simulink model "AssembledTEST1"  (R2016b)
settings: Solver=VariableStepAuto  StartTime=0.0  StopTime=60  RelTol=1e-3
values from neighbouring files (symbols this model uses):
  ail_data = [ ... (first row only)    [lookup_init.m]
  Ap = pi * (D^2)/4    (= 5.69167367599)    [constants_init.m]
  Aw = 10.0    (= 10)    [constants_init.m]
  b = 15.85    [constants_init.m]
  beta0_data = [ ... (first row only)    [lookup_init.m]
  c0 = 2.3774    [constants_init.m]
  c_i = 1.847    [constants_init.m]
  cdrag_data = [ ... (first row only)    [lookup_init.m]
  clean_wing_data = [ ... (first row only)    [lookup_init.m]
  crt = 1.6764    [constants_init.m]
  CT_data = [ ... (first row only)    [lookup_init.m]
  D = 2.692    [constants_init.m]
  D0q_10 = 0.0778    [constants_init.m]
  D0q_20 = 0.2634    [constants_init.m]
  D0q_35 = 0.7099    [constants_init.m]
  DCDi_data = [ ... (first row only)    [lookup_init.m]
  DCM0b = -0.188    [constants_init.m]
  Deh_f_on_data = [ ... (first row only)    [lookup_init.m]
  Deh_on_data = [ ... (first row only)    [lookup_init.m]
  df = 1.981    [constants_init.m]
  DOWN_0 = HP * F2M    (= 1830.0192)    [InitialiseJ31.m]    (also in Trim.m = -xtrim(12))
  Dqhq_data = [ ... (first row only)    [lookup_init.m]
  e0 = d2r(2.0)    [constants_init.m]
  e_data10 = [ ... (first row only)    [lookup_init.m]
  e_data20 = [ ... (first row only)    [lookup_init.m]
  e_data35 = [ ... (first row only)    [lookup_init.m]
  EAST_0 = 0.0    (= 0)    [InitialiseJ31.m]    (also in Trim.m = xtrim(11))
  elaw_0 = -7.50225e+2    (= -750.225)    [constants_init.m]
  elaw_1 = 8.98698    [constants_init.m]
  elaw_2 = -6.94240e-3    (= -0.0069424)    [constants_init.m]
  FLAP = 0    [InitialiseJ31.m]
  flaps_lift_data = [ ... (first row only)    [lookup_init.m]
  flaps_moment_data = [ ... (first row only)    [lookup_init.m]
  flaps_tail_data = [ ... (first row only)    [lookup_init.m]
  flaps_wing_data = [ ... (first row only)    [lookup_init.m]
  fmc_data = [ ... (first row only)    [lookup_init.m]
  fmf_data = [ ... (first row only)    [lookup_init.m]
  fmn_data = [ ... (first row only)    [lookup_init.m]
  fus_data = [ ... (first row only)    [lookup_init.m]
  gamma_t = 0.578    [constants_init.m]
  h_data10 = [ ... (first row only)    [lookup_init.m]
  h_data20 = [ ... (first row only)    [lookup_init.m]
  h_data35 = [ ... (first row only)    [lookup_init.m]
  INERTIA = [IXX,IXY,IXZ;IXY,IYY,IYZ;IXZ,IYZ,IZZ]    [InitialiseJ31.m]
  it = d2r(-2.3)    [constants_init.m]
  iw = d2r(1.33)    [constants_init.m]
  Iwn2 = 0.636    [constants_init.m]
  J_W = 1.26    [constants_init.m]
  K1_data = [ ... (first row only)    [lookup_init.m]
  k1f_data = [ ... (first row only)    [lookup_init.m]
  k_data = [ ... (first row only)    [lookup_init.m]
  L_r0_10f = -0.0096    [constants_init.m]
  L_r0_20f = -0.0180    (= -0.018)    [constants_init.m]
  L_r0_35f = -0.0245    [constants_init.m]
  l_t = 11.6205 - 5.6642    (= 5.9563)    [constants_init.m]
  ld_data = [ ... (first row only)    [lookup_init.m]
  Lt = 4.686    [constants_init.m]
  Lt_dash = 247.1 * 0.3048/12    (= 6.27634)    [constants_init.m]
  Lv_b = -0.00145    [constants_init.m]
  Lv_h = 0.0445    [constants_init.m]
  Lv_n = 0.0165    [constants_init.m]
  mac = 1.716    [constants_init.m]
  mach_ffr = 0.4158    [constants_init.m]
  mach_pow = 0.7984    [constants_init.m]
  n = 1591/60    (= 26.5166666667)    [constants_init.m]
  NORTH_0 = 0.0    (= 0)    [InitialiseJ31.m]    (also in Trim.m = xtrim(10))
  Nr_b = -0.0060    (= -0.006)    [constants_init.m]
  Nv_n = -0.0005    [constants_init.m]
  Nv_wb = -0.0719    [constants_init.m]
  P_0 = 0.0    (= 0)    [InitialiseJ31.m]    (also in Trim.m = xtrim(4))
  pdrag_data = [ ... (first row only)    [lookup_init.m]
  PHI_0 = xtrim(7)    [Trim.m]
  piAt = At * pi    (= 17.5929188601)    [constants_init.m]
  piAw = Aw * pi    (= 31.4159265359)    [constants_init.m]
  PSI_0 = xtrim(9)    [Trim.m]
  Q_0 = 0.0    (= 0)    [InitialiseJ31.m]    (also in Trim.m = xtrim(5))
  R2D = 180/pi    (= 57.2957795131)    [InitialiseJ31.m]
  R_0 = 0.0    (= 0)    [InitialiseJ31.m]    (also in Trim.m = xtrim(6))
  s_e = 0.0954    [constants_init.m]
  side_data = [ ... (first row only)    [lookup_init.m]
  sideforce_data = [ ... (first row only)    [lookup_init.m]
  Sit = 1.874    [constants_init.m]
  Sn = 0.552    [constants_init.m]
  Sref = (pi/4) * df^2    (= 3.08218592191)    [constants_init.m]
  St = 7.785    [constants_init.m]
  Sw = 25.084    [constants_init.m]
  tail_data = [ ... (first row only)    [lookup_init.m]
  THETA_0 = xtrim(8)    [Trim.m]
  U_0 = xtrim(1)    [Trim.m]
  upwash_clean = [ ... (first row only)    [lookup_init.m]
  upwash_flaps = [ ... (first row only)    [lookup_init.m]
  V_0 = xtrim(2)    [Trim.m]
  vortex_drag_factors = [ ... (first row only)    [lookup_init.m]
  W_0 = xtrim(3)    [Trim.m]
  X_ci = ((223 - 140)*0.3048/12) - Xp_dash    (= 0.09144)    [constants_init.m]
  xacf = -6.653    [constants_init.m]
  xacn = (223 - 197.3)*0.3048/12    (= 0.65278)    [constants_init.m]
  xb0 = c0 * xb0_c0    (= 0.5895952)    [constants_init.m]
  xcit = -l_t - ycit * sin(d2r(11.31)) - (0.981/4)    [constants_init.m]
  Xp_dash = 79.4  * 0.3048/12    (= 2.01676)    [constants_init.m]
  xyz_p = [140.0*0.3048/12;-107.0*0.3048/12;11.5*0.3048/12]    [constants_init.m]
  xyz_s = [140.0*0.3048/12; 107.0*0.3048/12;11.5*0.3048/12]    [constants_init.m]
  ycit = 2.306    [constants_init.m]
  Yr_b = -0.0283    [constants_init.m]
  Yv_n = -0.0458    [constants_init.m]
  Yv_wb = -0.2627    [constants_init.m]
  Z_ht = 11.5*0.3048/12 - zact    (= 1.7271)    [constants_init.m]
  zacf = -1.741    [constants_init.m]
  zacn = 11.5*0.3048/12    (= 0.2921)    [constants_init.m]
  zact = -1.435    [constants_init.m]
  zacw = 0.929 - (3.307 * tan(d2r(7)))    [constants_init.m]
  Zt_dash = 12.0  * 0.3048/12    (= 0.3048)    [constants_init.m]
undefined symbols (not defined in the file or in its folder): CG, MASS
libraries: aerolibasang x3, aerolibatmos2 x1
(part 2 of 5)

== system AssembledTEST1/Subsystem/Longitudinal Aerodynamics/Get Nacelles XZM ==
  In2 : Inport
  In1 : Inport  Port=2
  Bus Selector : BusSelector  OutputSignals=alpha_b,q_bar,Flap,Mach
  Constant : Constant  Value=xacn
  Constant1 : Constant  Value=zacn
  Constant2 : Constant  Value=0
  Constant6 : Constant  Value=mac
  Constant7 : Constant  Value=Sw
  Get XZM : Subsystem
      mask Display:
      | port_label('input',1,'lift [N]')
      | port_label('input',2,'drag [N]')
      | port_label('input',3,'\alpha [rad]','texmode','on')
      | port_label('input',4,'M [Nm]','texmode','on')
      | port_label('input',5,'x_{ac} [m]','texmode','on')
      | port_label('input',6,'z_{ac} [m]','texmode','on')
      | port_label('output',1,'X [N]')
      | port_label('output',2,'Z [N]')
      | port_label('output',3,'M [Nm]')
  Product7 : Product  Inputs=5  RndMeth=Zero
  Subsystem : Subsystem
      mask Display:
      | port_label('output',1,'(C_{m\alpha})_{n(\epsilon)}','texmode','on')
      | port_label('input',1,'Flap')
      | port_label('input',2,'Mach')
  Out1 : Outport
  Out2 : Outport  Port=2
  Out3 : Outport  Port=3
  wires:
  Get XZM/1(X) -> Out1/1
  In1/1 -> Get XZM/2(D)
  Get XZM/2(Z) -> Out2/1
  Get XZM/3(M) -> Out3/1
  Constant1/1 -> Get XZM/6(z)
  Constant/1 -> Get XZM/5(x)
  In2/1 -> Bus Selector/1
  Bus Selector/1 -> Get XZM/3(alpha), Product7/1  "<alpha_b>"
  Constant6/1 -> Product7/2
  Constant7/1 -> Product7/3
  Constant2/1 -> Get XZM/1(L)
  Bus Selector/2 -> Product7/4  "<q_bar>"
  Bus Selector/3 -> Subsystem/1(In2)  "<Flap>"
  Bus Selector/4 -> Subsystem/2(In1)  "<Mach>"
  Subsystem/1(Out1) -> Product7/5
  Product7/1 -> Get XZM/4(M0)

== system AssembledTEST1/Subsystem/Longitudinal Aerodynamics/Get Tail XZM ==
  In1 : Inport
  In2 : Inport  Port=2
  In3 : Inport  Port=3
  In4 : Inport  Port=4
  In5 : Inport  Port=5
  Bus Selector : BusSelector  OutputSignals=Mach,q_bar,Elevator
  Constant1 : Constant  Value=-0.652
  Constant13 : Constant  Value=zact
  Constant2 : Constant  Value=Sw
  Constant3 : Constant  Value=mac
  Get XZM : Subsystem
      mask Display:
      | port_label('input',1,'lift [N]')
      | port_label('input',2,'drag [N]')
      | port_label('input',3,'\alpha [rad]','texmode','on')
      | port_label('input',4,'M_0 [Nm]','texmode','on')
      | port_label('input',5,'x_{ac} [m]','texmode','on')
      | port_label('input',6,'z_{ac} [m]','texmode','on')
      | port_label('output',1,'X [N]')
      | port_label('output',2,'Z [N]')
      | port_label('output',3,'M [Nm]')
  Product1 : Product  Inputs=6  RndMeth=Zero
  get kf : Lookup  InputValues=tail_data(:,1)  Table=tail_data(:,6)
  Out1 : Outport
  Out2 : Outport  Port=2
  Out3 : Outport  Port=3
  wires:
  Constant13/1 -> Get XZM/6(z)
  In1/1 -> Get XZM/1(L)
  Get XZM/1(X) -> Out1/1
  In2/1 -> Get XZM/2(D)
  In3/1 -> Get XZM/3(alpha)
  Get XZM/2(Z) -> Out2/1
  In5/1 -> Get XZM/5(x)
  Get XZM/3(M) -> Out3/1
  In4/1 -> Bus Selector/1
  Bus Selector/1 -> get kf/1  "<Mach>"
  get kf/1 -> Product1/1
  Bus Selector/2 -> Product1/2  "<q_bar>"
  Bus Selector/3 -> Product1/3  "<Elevator>"
  Constant1/1 -> Product1/4
  Constant2/1 -> Product1/5
  Constant3/1 -> Product1/6
  Product1/1 -> Get XZM/4(M0)

== system AssembledTEST1/Subsystem/Longitudinal Aerodynamics/Get Wing & Tail Lift ==
  Flap : Inport
  Mach : Inport  Port=2
  V : Inport  Port=3
  aoa : Inport  Port=4
  qbar : Inport  Port=5
  q : Inport  Port=6
  xcg : Inport  Port=7
  wdot : Inport  Port=8
  Elevator : Inport  Port=9
  Constant : Constant
  Terminator{,1..3} (4 alike) : Terminator
  get_tail_lift : Subsystem
      mask help:
      | This subsystem determines the lift and angle of attack for the tailplane at the cacluated wing angle of attack (aoa_w)  and Mach Number for the given Elevator angle. Uses the method given in ESDU 80020 and ESDU 89029. It includes modification of the incidence with pitch rate and vertical acceleration.
      |
      | Author: A Cooke Date: 24 Mar 05, modified 29 Mar 05, 8 Mar 07, 12 Sep 07
  get_wing_lift : Subsystem
      mask help:
      | This subsystem determines the lift for the wing/body combination at the specified body angle of attack (aoa), Mach Number and dynamic pressure  (qbar) for the given flap setting (Flap). Uses the method given in ESDU 96003.  It includes modification of the incidence with pitch rate.
      |
      | Author: A Cooke Date: 23 Feb 05, modified 29 Mar 05, 1 Aug 06, 8 Mar 07
  get_wing_lift_basic : Subsystem
      mask help:
      | This subsystem determines the lift for the wing/body combination at the specified body angle of attack (aoa), Mach Number and dynamic pressure  (qbar) for the given flap setting (Flap). Uses the method given in ESDU 96003.  It includes modification of the incidence with pitch rate.
      |
      | Author: A Cooke Date: 23 Feb 05, modified 29 Mar 05, 1 Aug 06, 8 Mar 07
  wng_lift : Outport
  CLw : Outport  Port=2
  aoa_w : Outport  Port=3
  xac_w : Outport  Port=4
  CLt : Outport  Port=5
  tail_lift : Outport  Port=6
  aoa_t : Outport  Port=7
  a1t : Outport  Port=8
  downwash : Outport  Port=9
  xac_t : Outport  Port=10
  CLb : Outport  Port=11
  alpha0 : Outport  Port=12
  wires:
  Flap/1 -> get_wing_lift/1(Flap), get_tail_lift/11(Flap)
  Mach/1 -> get_tail_lift/1(Mach), get_wing_lift_basic/2(Mach), get_wing_lift/2(Mach)
  V/1 -> get_wing_lift/3(V), get_tail_lift/3(V), get_wing_lift_basic/3(V)
  aoa/1 -> get_wing_lift/4(aoa), get_wing_lift_basic/4(aoa)
  qbar/1 -> get_wing_lift/5(qbar), get_tail_lift/2(qbar), get_wing_lift_basic/5(qbar)
  get_wing_lift/1(wing_lift) -> wng_lift/1
  q/1 -> get_wing_lift/6(q), get_tail_lift/4(q), get_wing_lift_basic/6(q)
  xcg/1 -> get_wing_lift/7(xcg), get_tail_lift/5(xcg), get_wing_lift_basic/7(xcg)
  get_wing_lift/2(CL) -> CLw/1
  get_wing_lift/3(aoa_w) -> aoa_w/1, get_tail_lift/6(aoa_w)
  get_wing_lift/4(alpha0) -> get_tail_lift/9(alpha0), alpha0/1
  get_tail_lift/1(aoa_t) -> aoa_t/1
  get_tail_lift/2(CLt) -> CLt/1
  get_tail_lift/3(tail_lift) -> tail_lift/1
  wdot/1 -> get_tail_lift/7(wdot)
  Elevator/1 -> get_tail_lift/8(Elevator)
  get_tail_lift/4(a1t) -> a1t/1
  get_tail_lift/5(e) -> downwash/1
  get_tail_lift/6(xac_t) -> xac_t/1
  get_wing_lift/5(xac_w) -> get_tail_lift/10(xac_w), xac_w/1
  Constant/1 -> get_wing_lift_basic/1(Flap)
  get_wing_lift_basic/1(wing_lift) -> Terminator/1
  get_wing_lift_basic/2(CL) -> CLb/1
  get_wing_lift_basic/3(aoa_w) -> Terminator1/1
  get_wing_lift_basic/4(alpha0) -> Terminator2/1
  get_wing_lift_basic/5(xac_w) -> Terminator3/1

== system AssembledTEST1/Subsystem/Longitudinal Aerodynamics/Get Wing XZM ==
  In1 : Inport
  In2 : Inport  Port=2
  In3 : Inport  Port=3
  In4 : Inport  Port=4
  In5 : Inport  Port=5
  Bus Selector3 : BusSelector  OutputSignals=Mach,Flap,q_bar
  Constant9 : Constant  Value=zacw
  Get XZM : Subsystem
      mask Display:
      | port_label('input',1,'drag [N]')
      | port_label('input',2,'lift [N]')
      | port_label('input',3,'\alpha [rad]','texmode','on')
      | port_label('input',4,'M_0 [Nm]','texmode','on')
      | port_label('input',5,'x_{ac} [m]','texmode','on')
      | port_label('input',6,'z_{ac} [m]','texmode','on')
      | port_label('output',1,'X [N]')
      | port_label('output',2,'Z [N]')
      | port_label('output',3,'M [Nm]')
  get_M0w : Subsystem
  Out1 : Outport
  Out2 : Outport  Port=2
  Out3 : Outport  Port=3
  wires:
  Bus Selector3/3 -> get_M0w/3(qbar)  "<q_bar>"
  Bus Selector3/2 -> get_M0w/2(Flap)  "<Flap>"
  Bus Selector3/1 -> get_M0w/1(Mach)  "<Mach>"
  get_M0w/1(M0) -> Get XZM/4(M0)
  Constant9/1 -> Get XZM/6(z)
  In3/1 -> Get XZM/3(alpha)
  In1/1 -> Get XZM/1(D)
  Get XZM/1(X) -> Out1/1
  In2/1 -> Get XZM/2(L)
  Get XZM/2(Z) -> Out2/1
  In4/1 -> Bus Selector3/1
  In5/1 -> Get XZM/5(x)
  Get XZM/3(M) -> Out3/1

== system AssembledTEST1/Subsystem/Longitudinal Aerodynamics/get_CDvwbasic ==
  aoa_w : Inport
  flap : Inport  Port=2
  CLw : Inport  Port=3
  Mach : Inport  Port=4
  Add4 : Sum  Inputs=+++
  Constant2 : Constant  Value=piAw
  Divide : Product  Inputs=*/
  Fcn1 : Fcn  Expr=u(1)^2
  Fcn2 : Fcn  Expr=u(1)^2
  Product3 : Product  RndMeth=Zero
  Product4 : Product  RndMeth=Zero
  Product5 : Product  Inputs=3  RndMeth=Zero
  get_CL1 : Sum  Inputs=+-
  get_DelCL0tw : Subsystem
  get_k1 : Lookup2D  RowIndex=aw_ords  ColumnIndex=Mach_ords  Table=k_data
  get_k1f : Lookup  InputValues=k1f_data(:,1)  Table=k1f_data(:,2)
  get_kf : Subsystem
  r2d : Gain  Gain=180/pi
  CDvw : Outport
  wires:
  get_DelCL0tw/1(DelCL0tw) -> get_CL1/2, Fcn2/1, Product5/2
  get_CL1/1 -> Fcn1/1, Product5/3
  Fcn2/1 -> Product3/1
  get_kf/1(kf) -> Product3/2
  Fcn1/1 -> Product4/1
  get_k1/1 -> Product4/2
  get_k1f/1 -> Product5/1
  Product5/1 -> Add4/1
  Product4/1 -> Add4/2
  Product3/1 -> Add4/3
  Add4/1 -> Divide/1
  Constant2/1 -> Divide/2
  flap/1 -> get_DelCL0tw/1(flap), get_kf/1(flap)
  Mach/1 -> get_DelCL0tw/2(Mach), get_kf/2(Mach), get_k1/2
  aoa_w/1 -> get_k1f/1, r2d/1
  Divide/1 -> CDvw/1
  CLw/1 -> get_CL1/1
  r2d/1 -> get_k1/1

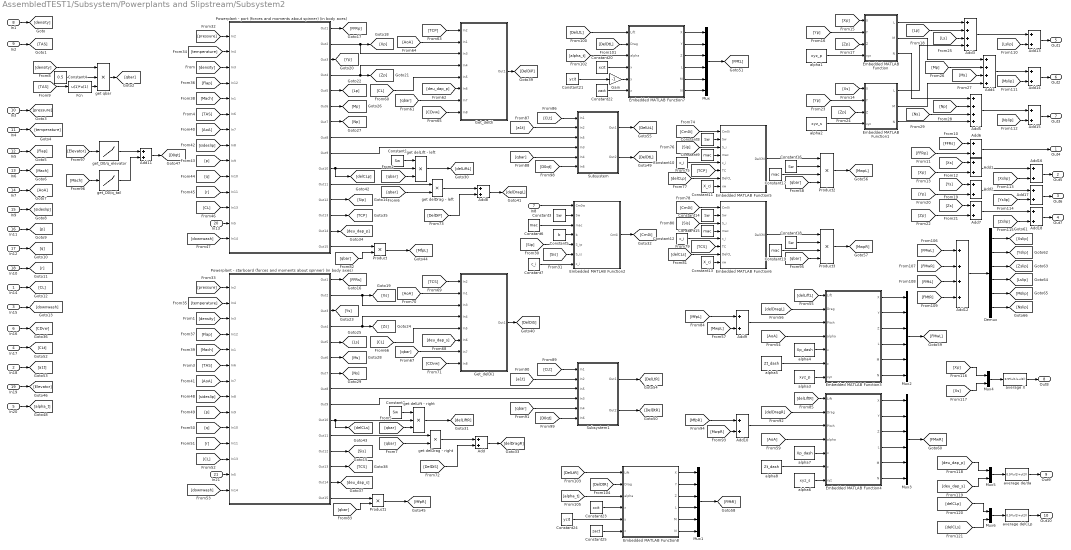
== system AssembledTEST1/Subsystem/Powerplants and Slipstream/Subsystem2 ==
  In14 : Inport
  In18 : Inport  Port=2
  In15 : Inport  Port=3
  In17 : Inport  Port=4
  In20 : Inport  Port=5
  In16 : Inport  Port=6
  In8 : Inport  Port=7
  In1 : Inport  Port=8
  In2 : Inport  Port=9
  In3 : Inport  Port=10
  In4 : Inport  Port=11
  In5 : Inport  Port=12
  In6 : Inport  Port=13
  In7 : Inport  Port=14
  In9 : Inport  Port=15
  In11 : Inport  Port=16
  In12 : Inport  Port=17
  In10 : Inport  Port=18
  In19 : Inport  Port=19
  In13 : Inport  Port=20
  In21 : Inport  Port=21
  Add{,1..2,6..11,13..18} (15 alike) : Sum
  Add{3..5,12} (4 alike) : Sum  Inputs=++++
  Constant{1..3,8,14,16,18} (7 alike) : Constant  Value=Sw
  Constant10 : Constant  Value=c_i
  Constant11 : Constant  Value=X_ci
  Constant12 : Constant  Value=c_i
  Constant13 : Constant  Value=X_ci
  Constant{6,9,15,17,19} (5 alike) : Constant  Value=mac
  Constant20 : Constant  Value=xcit
  Constant21 : Constant  Value=ycit
  Constant22 : Constant  Value=zact
  Constant23 : Constant  Value=xcit
  Constant24 : Constant  Value=ycit
  Constant25 : Constant  Value=zact
  Constant4 : Constant  Value=0.5
  Constant5 : Constant  Value=b
  Constant7 : Constant  Value=c_i
  Demux : Demux  Outputs=6
  Embedded MATLAB Function : MATLAB Function  TreatAsAtomicUnit=on
  Embedded MATLAB Function1 : MATLAB Function  TreatAsAtomicUnit=on
  Embedded MATLAB Function2 : MATLAB Function  TreatAsAtomicUnit=on
  Embedded MATLAB Function3 : MATLAB Function  TreatAsAtomicUnit=on
  Embedded MATLAB Function4 : MATLAB Function  TreatAsAtomicUnit=on
  Embedded MATLAB Function5 : MATLAB Function  TreatAsAtomicUnit=on
  Embedded MATLAB Function6 : MATLAB Function  TreatAsAtomicUnit=on
  Embedded MATLAB Function7 : MATLAB Function  TreatAsAtomicUnit=on
  Embedded MATLAB Function8 : MATLAB Function  TreatAsAtomicUnit=on
  Fcn : Fcn  Expr=u(1)*u(1)
  Gain : Gain  Gain=-1
  Get_delDi : Subsystem
      mask Display:
      | port_label('output',1,'\DeltaD_i','texmode','on')
      | port_label('input',2,'\alpha_b','texmode','on')
      | port_label('input',3,'X_p','texmode','on')
      | port_label('input',4,'Z_p','texmode','on')
      | port_label('input',5,'C_{Lw}','texmode','on')
      | port_label('input',6,'\partial\epsilon_u/\partial\alpha_p','texmode','on')
      | port_label('input',7,'q_\infty','texmode','on')
      | port_label('input',8,'(C_{Di})_w','texmode','on')
      | port_label('input',1,'S_wT_C/8R^2_p','texmode','on')
      | text(0.5,0.5,'Get\DeltaD_i','texmode','on')
  Get_delDi1 : Subsystem
      mask Display:
      | port_label('output',1,'\DeltaD_i','texmode','on')
      | port_label('input',2,'\alpha_b','texmode','on')
      | port_label('input',3,'X_p','texmode','on')
      | port_label('input',4,'Z_p','texmode','on')
      | port_label('input',5,'C_{Lw}','texmode','on')
      | port_label('input',6,'\partial\epsilon_u/\partial\alpha_p','texmode','on')
      | port_label('input',7,'q_\infty','texmode','on')
      | port_label('input',8,'(C_{Di})_w','texmode','on')
      | port_label('input',1,'S_wT_C/8R^2_p','texmode','on')
      | text(0.5,0.5,'Get\DeltaD_i','texmode','on')
  Mux{,1..3} (4 alike) : Mux  Inputs=6
  Mux4 : Mux  Inputs=2
  Mux5 : Mux  Inputs=2
  Mux6 : Mux  Inputs=2
  Powerplant - port (forces and moments about spinner) (in body axes) : Subsystem
      mask Display:
      | port_label('output',1,'FFR [kg/h]')
      | port_label('output',2,'X [N]')
      | port_label('output',3,'Y [N]')
      | port_label('output',4,'Z [N]')
      | port_label('output',5,'L [Nm]')
      | port_label('output',6,'M [Nm]')
      | port_label('output',7,'N [Nm]')
      | port_label('output',8,'\Deltaq_h/q_\infty','texmode','on')
      | port_label('output',9,'(\Delta\epsilon_h)_{power} [rad]','texmode','on')
      | port_label('output',10,'(\DeltaC_{Lw})_{slip}','texmode','on')
      | port_label('output',11,'\Delta(D_{0w}/q)_{slip}','texmode','on')
      | port_label('output',12,'S_i [m^2]','texmode','on')
      | port_label('output',13,'S_wT_C/8R^2_p','texmode','on')
      | port_label('output',14,'\partial\epsilon_u/\partial\alpha_p','texmode','on')
      | port_label('output',15,'\DeltaM_p/q_\infty','texmode','on')
      | port_label('input',1,'P_\infty [N/m^2]','texmode','on')
      | port_label('input',3,'\rho_\infty [kg/m^3]','texmode','on')
      | port_label('input',2,'T_\infty [K]','texmode','on')
      | port_label('input',4,'Flap')
      | port_label('input',6,'V [m/s]')
      | port_label('input',7,'\alpha_b [rad]','texmode','on')
      | port_label('input',8,'\beta [rad]','texmode','on')
      | port_label('input',9,'p [rad/s]')
      | port_label('input',10,'q [rad/s]')
      | port_label('input',11,'r [rad/s]')
      | port_label('input',5,'Mach')
      | port_label('input',12,'C_{Lw}','texmode','on')
      | port_label('input',13,'Throttle [%]')
      | port_label('input',14,'\epsilon_h [rad]','texmode','on')
  Powerplant - starboard (forces and moments about spinner) (in body axes) : Subsystem
      mask Display:
      | port_label('output',1,'FFR [kg/h]')
      | port_label('output',2,'X [N]')
      | port_label('output',3,'Y [N]')
      | port_label('output',4,'Z [N]')
      | port_label('output',5,'L [Nm]')
      | port_label('output',6,'M [Nm]')
      | port_label('output',7,'N [Nm]')
      | port_label('output',8,'\Deltaq_h/q_\infty','texmode','on')
      | port_label('output',9,'(\Delta\epsilon_h)_{power} [rad]','texmode','on')
      | port_label('output',10,'(\DeltaC_{Lw})_{slip}','texmode','on')
      | port_label('output',12,'S_i [m^2]','texmode','on')
      | port_label('output',11,'\Delta(D_{0w}/q)_{slip}','texmode','on')
      | port_label('output',13,'S_wT_C/8R^2_p','texmode','on')
      | port_label('output',14,'\partial\epsilon_u/\partial\alpha_p','texmode','on')
      | port_label('output',15,'\DeltaM_p/q_\infty','texmode','on')
      | port_label('input',1,'P_\infty [N/m^2]','texmode','on')
      | port_label('input',3,'\rho_\infty [kg/m^3]','texmode','on')
      | port_label('input',2,'T_\infty [K]','texmode','on')
      | port_label('input',4,'Flap')
      | port_label('input',6,'V [m/s]')
      | port_label('input',7,'\alpha_b [rad]','texmode','on')
      | port_label('input',8,'\beta [rad]','texmode','on')
      | port_label('input',9,'p [rad/s]')
      | port_label('input',10,'q [rad/s]')
      | port_label('input',11,'r [rad/s]')
      | port_label('input',5,'Mach')
      | port_label('input',12,'C_{Lw}','texmode','on')
      | port_label('input',13,'Throttle [%]')
      | port_label('input',14,'\epsilon_h [rad]','texmode','on')
  Product : Product  RndMeth=Zero
  Product1 : Product  RndMeth=Zero
  Product2 : Product  Inputs=4  RndMeth=Zero
  Product3 : Product  Inputs=4  RndMeth=Zero
  Subsystem : Subsystem
      mask Display:
      | port_label('input',1,'C_{Lt}','texmode','on')
      | port_label('input',2,'a_{1t}','texmode','on')
      | port_label('input',4,'(\Delta\epsilon_{h})_{power}','texmode','on')
      | port_label('input',3,'\Deltaq_h/q_\infty','texmode','on')
      | port_label('input',5,'q_\infty','texmode','on')
      | port_label('output',1,'\DeltaL_t','texmode','on')
      | port_label('input',6,'(D_0/q_\infty)_t','texmode','on')
      | port_label('output',2,'\DeltaD_t','texmode','on')
  Subsystem1 : Subsystem
      mask Display:
      | port_label('input',1,'C_{Lt}','texmode','on')
      | port_label('input',2,'a_{1t}','texmode','on')
      | port_label('input',4,'(\Delta\epsilon_{h})_{power}','texmode','on')
      | port_label('input',3,'\Deltaq_h/q_\infty','texmode','on')
      | port_label('input',5,'q_\infty','texmode','on')
      | port_label('output',1,'\DeltaL_t','texmode','on')
      | port_label('input',6,'(D_0/q_\infty)_t','texmode','on')
      | port_label('output',2,'\DeltaD_t','texmode','on')
  alpha1 : Constant  Value=xyz_p
  alpha2 : Constant  Value=xyz_s
  alpha3 : Constant  Value=xyz_p
  alpha4 : Constant  Value=Xp_dash
  alpha5 : Constant  Value=Zt_dash
  alpha6 : Constant  Value=xyz_s
  alpha7 : Constant  Value=Xp_dash
  alpha8 : Constant  Value=Zt_dash
  average X : Fcn  Expr=0.5*(u(1)+u(2))
  average de/da : Fcn  Expr=0.5*(u(1)+u(2))
  average delCLp : Fcn  Expr=0.5*(u(1)+u(2))
  get delDrag - left : Product  RndMeth=Zero
  get delDrag - right : Product  RndMeth=Zero
  get delLift - left : Product  Inputs=3  RndMeth=Zero
  get delLift - right : Product  Inputs=3  RndMeth=Zero
  get qbar : Product  Inputs=3  RndMeth=Zero
  get_D0/q_elevator : Lookup  InputValues=cdrag_data(:,1)  Table=cdrag_data(:,2)
  get_D0/q_tail : Lookup  InputValues=pdrag_data(:,1)  Table=pdrag_data(:,4)
  Out4 : Outport
  Out5 : Outport  Port=2
  Out6 : Outport  Port=3
  Out7 : Outport  Port=4
  Out1 : Outport  Port=5
  Out2 : Outport  Port=6
  Out3 : Outport  Port=7
  Out8 : Outport  Port=8
  Out9 : Outport  Port=9
  Out10 : Outport  Port=10
  wires:
  [density] -> Powerplant - port (forces and moments about spinner) (in body axes)/3(In3)
  [density] -> Powerplant - starboard (forces and moments about spinner) (in body axes)/3(In3)
  [TAS] -> Powerplant - starboard (forces and moments about spinner) (in body axes)/6(In6)
  [TAS] -> Powerplant - port (forces and moments about spinner) (in body axes)/6(In6)
  In13/1 -> Powerplant - port (forces and moments about spinner) (in body axes)/13(In5)
  In21/1 -> Powerplant - starboard (forces and moments about spinner) (in body axes)/13(In5)
  alpha1/1 -> Embedded MATLAB Function/4(xyz)
  alpha2/1 -> Embedded MATLAB Function1/4(xyz)
  Embedded MATLAB Function/1(L) -> Add3/1
  [density] -> get qbar/1
  Constant4/1 -> get qbar/2
  get qbar/1 -> [qbar]
  Constant1/1 -> get delLift - left/1
  [qbar] -> get delLift - left/3
  Constant2/1 -> get delLift - right/1
  [qbar] -> get delLift - right/3
  Constant3/1 -> Embedded MATLAB Function2/2(Sw)
  Constant5/1 -> Embedded MATLAB Function2/4(b)
  Constant6/1 -> Embedded MATLAB Function2/3(mac)
  Constant7/1 -> Embedded MATLAB Function2/7(c_i)
  Powerplant - port (forces and moments about spinner) (in body axes)/12(Out12) -> [Sip]
  Powerplant - starboard (forces and moments about spinner) (in body axes)/12(Out12) -> [Sis]
  Powerplant - starboard (forces and moments about spinner) (in body axes)/1(Out1) -> [FFRs]
  Powerplant - port (forces and moments about spinner) (in body axes)/1(Out1) -> [FFRp]
  [FFRs] -> Add6/1
  [FFRp] -> Add6/2
  Powerplant - port (forces and moments about spinner) (in body axes)/2(Out2) -> [Xp], Get_delDi/3(In3)
  Powerplant - starboard (forces and moments about spinner) (in body axes)/2(Out2) -> [Xs], Get_delDi1/3(In3)
  [Xp] -> Add1/2
  [Xs] -> Add1/1
  [Xs] -> Embedded MATLAB Function1/1(X)
  [Xp] -> Embedded MATLAB Function/1(X)
  Embedded MATLAB Function1/1(L) -> Add3/4
  Embedded MATLAB Function1/3(N) -> Add5/4
  Embedded MATLAB Function/3(N) -> Add5/1
  Embedded MATLAB Function/2(M) -> Add4/1
  Embedded MATLAB Function1/2(M) -> Add4/4
  Powerplant - port (forces and moments about spinner) (in body axes)/3(Out3) -> [Yp]
  Powerplant - port (forces and moments about spinner) (in body axes)/4(Out4) -> [Zp], Get_delDi/4(In4)
  Powerplant - port (forces and moments about spinner) (in body axes)/5(Out5) -> [Lp]
  [Yp] -> Embedded MATLAB Function/2(Y)
  [Zp] -> Embedded MATLAB Function/3(Z)
  [Lp] -> Add3/2
  [Yp] -> Add2/2
  [Ys] -> Add2/1
  Powerplant - starboard (forces and moments about spinner) (in body axes)/3(Out3) -> [Ys]
  Powerplant - starboard (forces and moments about spinner) (in body axes)/4(Out4) -> [Zs], Get_delDi1/4(In4)
  Powerplant - starboard (forces and moments about spinner) (in body axes)/5(Out5) -> [Ls]
  [Zp] -> Add7/2
  [Zs] -> Add7/1
  [Yp] -> Embedded MATLAB Function1/2(Y)
  [Zp] -> Embedded MATLAB Function1/3(Z)
  [Ls] -> Add3/3
  Powerplant - port (forces and moments about spinner) (in body axes)/6(Out6) -> [Mp]
  Powerplant - port (forces and moments about spinner) (in body axes)/7(Out7) -> [Np]
  [Mp] -> Add4/2
  Powerplant - starboard (forces and moments about spinner) (in body axes)/6(Out6) -> [Ms]
  Powerplant - starboard (forces and moments about spinner) (in body axes)/7(Out7) -> [Ns]
  [Ms] -> Add4/3
  [Np] -> Add5/2
  [Ns] -> Add5/3
  [Sip] -> Embedded MATLAB Function2/5(S_ip)
  [Sis] -> Embedded MATLAB Function2/6(S_is)
  [pressure] -> Powerplant - port (forces and moments about spinner) (in body axes)/1(In2)
  [pressure] -> Powerplant - starboard (forces and moments about spinner) (in body axes)/1(In2)
  [temperature] -> Powerplant - port (forces and moments about spinner) (in body axes)/2(In4)
  [temperature] -> Powerplant - starboard (forces and moments about spinner) (in body axes)/2(In4)
  [Flap] -> Powerplant - port (forces and moments about spinner) (in body axes)/4(In12)
  [Flap] -> Powerplant - starboard (forces and moments about spinner) (in body axes)/4(In12)
  [Mach] -> Powerplant - port (forces and moments about spinner) (in body axes)/5(In1)
  [Mach] -> Powerplant - starboard (forces and moments about spinner) (in body axes)/5(In1)
  [AoA] -> Powerplant - port (forces and moments about spinner) (in body axes)/7(In7)
  [AoA] -> Powerplant - starboard (forces and moments about spinner) (in body axes)/7(In7)
  [sideslip] -> Powerplant - port (forces and moments about spinner) (in body axes)/8(In8)
  [p] -> Powerplant - port (forces and moments about spinner) (in body axes)/9(In9)
  [q] -> Powerplant - port (forces and moments about spinner) (in body axes)/10(In10)
  [r] -> Powerplant - port (forces and moments about spinner) (in body axes)/11(In11)
  [CL] -> Powerplant - port (forces and moments about spinner) (in body axes)/12(In13)
  [downwash] -> Powerplant - port (forces and moments about spinner) (in body axes)/14(In14)
  [sideslip] -> Powerplant - starboard (forces and moments about spinner) (in body axes)/8(In8)
  [p] -> Powerplant - starboard (forces and moments about spinner) (in body axes)/9(In9)
  [q] -> Powerplant - starboard (forces and moments about spinner) (in body axes)/10(In10)
  [r] -> Powerplant - starboard (forces and moments about spinner) (in body axes)/11(In11)
  [CL] -> Powerplant - starboard (forces and moments about spinner) (in body axes)/12(In13)
  [downwash] -> Powerplant - starboard (forces and moments about spinner) (in body axes)/14(In14)
  In8/1 -> Embedded MATLAB Function2/1(Cm0w)
  Powerplant - port (forces and moments about spinner) (in body axes)/10(Out10) -> get delLift - left/2, [delCLp]
  Powerplant - starboard (forces and moments about spinner) (in body axes)/10(Out10) -> get delLift - right/2, [delCLs]
  Powerplant - port (forces and moments about spinner) (in body axes)/11(Out11) -> get delDrag - left/1
  [qbar] -> get delDrag - left/2
  [qbar] -> get delDrag - right/2
  Powerplant - starboard (forces and moments about spinner) (in body axes)/11(Out11) -> get delDrag - right/1
  get delLift - left/1 -> [delLiftL]
  get delLift - right/1 -> [delLiftR]
  get delDrag - left/1 -> Add8/1
  [AoA] -> Embedded MATLAB Function3/4(alpha)
  alpha3/1 -> Embedded MATLAB Function3/7(xyz)
  [delDragL] -> Embedded MATLAB Function3/2(Drag)
  alpha4/1 -> Embedded MATLAB Function3/5(x)
  alpha5/1 -> Embedded MATLAB Function3/6(z)
  [TAS] -> Fcn/1
  Fcn/1 -> get qbar/3
  [CL] -> Get_delDi/5(In5)
  Powerplant - port (forces and moments about spinner) (in body axes)/14(Out14) -> [deu_dap_p]
  Powerplant - port (forces and moments about spinner) (in body axes)/13(Out13) -> [TCP]
  [qbar] -> Get_delDi/7(In7)
  [deu_dap_p] -> Get_delDi/6(In6)
  [TCP] -> Get_delDi/1(In2)
  [AoA] -> Get_delDi/2(In1)
  [CDvw] -> Get_delDi/8(In8)
  Powerplant - starboard (forces and moments about spinner) (in body axes)/13(Out13) -> [TCS]
  Powerplant - starboard (forces and moments about spinner) (in body axes)/14(Out14) -> [deu_dap_s]
  [CL] -> Get_delDi1/5(In5)
  [qbar] -> Get_delDi1/7(In7)
  [deu_dap_s] -> Get_delDi1/6(In6)
  [TCS] -> Get_delDi1/1(In2)
  [AoA] -> Get_delDi1/2(In1)
  [CDvw] -> Get_delDi1/8(In8)
  Get_delDi/1(Out1) -> [DelDiP]
  Get_delDi1/1(Out1) -> [DelDiS]
  get delDrag - right/1 -> Add/1
  Add/1 -> [delDragR]
  [DelDiS] -> Add/2
  Add8/1 -> [delDragL]
  [DelDiP] -> Add8/2
  Embedded MATLAB Function2/1(Cm0i) -> [Cm0i]
  [Cm0i] -> Embedded MATLAB Function5/1(Cm0i)
  Constant8/1 -> Embedded MATLAB Function5/2(Sw)
  Constant9/1 -> Embedded MATLAB Function5/4(mac)
  Constant10/1 -> Embedded MATLAB Function5/5(c_i)
  [Sip] -> Embedded MATLAB Function5/3(S_i)
  [TCP] -> Embedded MATLAB Function5/6(TC)
  [delCLp] -> Embedded MATLAB Function5/7(DelCL)
  Constant11/1 -> Embedded MATLAB Function5/8(xw)
  [Cm0i] -> Embedded MATLAB Function6/1(Cm0i)
  Constant14/1 -> Embedded MATLAB Function6/2(Sw)
  Constant15/1 -> Embedded MATLAB Function6/4(mac)
  Constant12/1 -> Embedded MATLAB Function6/5(c_i)
  [Sis] -> Embedded MATLAB Function6/3(S_i)
  [TCS] -> Embedded MATLAB Function6/6(TC)
  [delCLs] -> Embedded MATLAB Function6/7(DelCL)
  Constant13/1 -> Embedded MATLAB Function6/8(xw)
  Powerplant - port (forces and moments about spinner) (in body axes)/15(Out15) -> Product/1
  [qbar] -> Product/2
  Product/1 -> [MfpL]
  Powerplant - starboard (forces and moments about spinner) (in body axes)/15(Out15) -> Product1/1
  [qbar] -> Product1/2
  Product1/1 -> [MfpR]
  Add9/1 -> Embedded MATLAB Function3/3(Pitch)
  [CLt] -> Subsystem/1(In1)
  [a1t] -> Subsystem/2(In2)
  Powerplant - port (forces and moments about spinner) (in body axes)/8(Out8) -> Subsystem/3(In5)
  Powerplant - port (forces and moments about spinner) (in body axes)/9(Out9) -> Subsystem/4(In3)
  [qbar] -> Subsystem/5(In4)
  Subsystem/1(Out1) -> [DelLtL]
  Embedded MATLAB Function5/1(DelCM) -> Product2/1
  Constant16/1 -> Product2/2
  Constant17/1 -> Product2/3
  [qbar] -> Product2/4
  Product2/1 -> [MwpL]
  Product3/1 -> [MwpR]
  [qbar] -> Product3/4
  Constant19/1 -> Product3/3
  Constant18/1 -> Product3/2
  Embedded MATLAB Function6/1(DelCM) -> Product3/1
  [delLiftL] -> Embedded MATLAB Function3/1(Lift)
  [MfpL] -> Add9/1
  [MwpL] -> Add9/2
  [AoA] -> Embedded MATLAB Function4/4(alpha)
  alpha6/1 -> Embedded MATLAB Function4/7(xyz)
  [delDragR] -> Embedded MATLAB Function4/2(Drag)
  alpha7/1 -> Embedded MATLAB Function4/5(x)
  alpha8/1 -> Embedded MATLAB Function4/6(z)
  Add10/1 -> Embedded MATLAB Function4/3(Pitch)
  [delLiftR] -> Embedded MATLAB Function4/1(Lift)
  [MfpR] -> Add10/1
  [MwpR] -> Add10/2
  get_D0/q_elevator/1 -> Add11/1
  get_D0/q_tail/1 -> Add11/2
  [Mach] -> get_D0/q_tail/1
  [Elevator] -> get_D0/q_elevator/1
  Add11/1 -> [D0qt]
  [D0qt] -> Subsystem/6(In6)
  Subsystem/2(Out2) -> [DelDtL]
  [CLt] -> Subsystem1/1(In1)
  Subsystem1/1(Out1) -> [DelLtR]
  Subsystem1/2(Out2) -> [DelDtR]
  [a1t] -> Subsystem1/2(In2)
  Powerplant - starboard (forces and moments about spinner) (in body axes)/8(Out8) -> Subsystem1/3(In5)
  Powerplant - starboard (forces and moments about spinner) (in body axes)/9(Out9) -> Subsystem1/4(In3)
  [qbar] -> Subsystem1/5(In4)
  [D0qt] -> Subsystem1/6(In6)
  [DelLtL] -> Embedded MATLAB Function7/1(Lift)
  [DelDtL] -> Embedded MATLAB Function7/2(Drag)
  [alpha_t] -> Embedded MATLAB Function7/3(alpha)
  Constant20/1 -> Embedded MATLAB Function7/4(x)
  Gain/1 -> Embedded MATLAB Function7/5(y)
  Constant21/1 -> Gain/1
  Constant22/1 -> Embedded MATLAB Function7/6(z)
  [DelLtR] -> Embedded MATLAB Function8/1(Lift)
  [DelDtR] -> Embedded MATLAB Function8/2(Drag)
  [alpha_t] -> Embedded MATLAB Function8/3(alpha)
  Constant23/1 -> Embedded MATLAB Function8/4(x)
  Constant24/1 -> Embedded MATLAB Function8/5(y)
  Constant25/1 -> Embedded MATLAB Function8/6(z)
  Embedded MATLAB Function7/1(X) -> Mux/1
  Embedded MATLAB Function7/2(Y) -> Mux/2
  Embedded MATLAB Function7/3(Z) -> Mux/3
  Embedded MATLAB Function7/4(L) -> Mux/4
  Embedded MATLAB Function7/5(M) -> Mux/5
  Embedded MATLAB Function7/6(N) -> Mux/6
  Mux/1 -> [FMtL]
  Embedded MATLAB Function8/1(X) -> Mux1/1
  Embedded MATLAB Function8/2(Y) -> Mux1/2
  Embedded MATLAB Function8/3(Z) -> Mux1/3
  Embedded MATLAB Function8/4(L) -> Mux1/4
  Embedded MATLAB Function8/5(M) -> Mux1/5
  Embedded MATLAB Function8/6(N) -> Mux1/6
  Mux1/1 -> [FMtR]
  Mux2/1 -> [FMwL]
  Embedded MATLAB Function3/1(X) -> Mux2/1
  Embedded MATLAB Function3/2(Y) -> Mux2/2
  Embedded MATLAB Function3/3(Z) -> Mux2/3
  Embedded MATLAB Function3/4(L) -> Mux2/4
  Embedded MATLAB Function3/5(M) -> Mux2/5
  Embedded MATLAB Function3/6(N) -> Mux2/6
  Mux3/1 -> [FMwR]
  Embedded MATLAB Function4/1(X) -> Mux3/1
  Embedded MATLAB Function4/2(Y) -> Mux3/2
  Embedded MATLAB Function4/3(Z) -> Mux3/3
  Embedded MATLAB Function4/4(L) -> Mux3/4
  Embedded MATLAB Function4/5(M) -> Mux3/5
  Embedded MATLAB Function4/6(N) -> Mux3/6
  [FMwL] -> Add12/1
  [FMwR] -> Add12/2
  [FMtL] -> Add12/3
  [FMtR] -> Add12/4
  Add12/1 -> Demux/1
  Demux/1 -> [Xslip]
  Demux/2 -> [Yslip]
  Demux/3 -> [Zslip]
  Demux/4 -> [Lslip]
  Demux/5 -> [Mslip]
  Demux/6 -> [Nslip]
  Add3/1 -> Add13/1
  [Lslip] -> Add13/2
  [Mslip] -> Add14/2
  Add4/1 -> Add14/1
  Add5/1 -> Add15/1
  [Nslip] -> Add15/2
  Add1/1 -> Add16/1
  [Xslip] -> Add16/2
  Add2/1 -> Add17/1
  [Yslip] -> Add17/2
  Add7/1 -> Add18/1
  [Zslip] -> Add18/2
  In1/1 -> [density]
  Add13/1 -> Out1/1
  In2/1 -> [TAS]
  Add14/1 -> Out2/1
  In3/1 -> [pressure]
  Add15/1 -> Out3/1
  In4/1 -> [temperature]
  Add6/1 -> Out4/1
  In5/1 -> [Flap]
  In6/1 -> [Mach]
  Add16/1 -> Out5/1
  In7/1 -> [AoA]
  Add17/1 -> Out6/1
  In9/1 -> [sideslip]
  Add18/1 -> Out7/1
  In11/1 -> [p]
  In12/1 -> [q]
  In10/1 -> [r]
  In14/1 -> [CL]
  In15/1 -> [downwash]
  In16/1 -> [CDvw]
  In17/1 -> [CLt]
  In18/1 -> [a1t]
  In19/1 -> [Elevator]
  In20/1 -> [alpha_t]
  Mux4/1 -> average X/1
  [Xp] -> Mux4/1
  [Xs] -> Mux4/2
  average X/1 -> Out8/1
  Mux5/1 -> average de/da/1
  [deu_dap_p] -> Mux5/1
  [deu_dap_s] -> Mux5/2
  average de/da/1 -> Out9/1
  average delCLp/1 -> Out10/1
  [delCLs] -> Mux6/2
  [delCLp] -> Mux6/1
  Mux6/1 -> average delCLp/1

== system AssembledTEST1/Subsystem/Powerplants and Slipstream/get_CM0 ==
  Mach : Inport
  Flap : Inport  Port=2
  Add : Sum
  Add1 : Sum
  Constant2 : Constant
  Constant3 : Constant  Value=0
  Multiport Switch : MultiPortSwitch  Inputs=4
  get_CM0W : Lookup  InputValues=clean_wing_data(:,1)  Table=clean_wing_data(:,7)
  get_delCM0a10 : Lookup  InputValues=flaps_moment_data(:,1)  Table=flaps_moment_data(:,2)
  get_delCM0a20 : Lookup  InputValues=flaps_moment_data(:,1)  Table=flaps_moment_data(:,3)
  get_delCM0a35 : Lookup  InputValues=flaps_moment_data(:,1)  Table=flaps_moment_data(:,4)
  CM0 : Outport
  wires:
  Mach/1 -> get_delCM0a35/1, get_delCM0a20/1, get_delCM0a10/1, get_CM0W/1
  Constant2/1 -> Add/1
  Add/1 -> Multiport Switch/1
  Constant3/1 -> Multiport Switch/2
  get_delCM0a10/1 -> Multiport Switch/3
  get_delCM0a20/1 -> Multiport Switch/4
  get_delCM0a35/1 -> Multiport Switch/5
  Flap/1 -> Add/2
  Multiport Switch/1 -> Add1/2
  Add1/1 -> CM0/1
  get_CM0W/1 -> Add1/1

== system AssembledTEST1/Subsystem/Lateral//Directional Aerodynamics/getYLN/Get_Lr_0_f ==
  In1 : Inport
  Add : Sum
  Constant1 : Constant  Value=0
  Constant10 : Constant
  Constant11 : Constant  Value=L_r0_10f
  Constant12 : Constant  Value=L_r0_20f
  Constant13 : Constant  Value=L_r0_35f
  Multiport Switch : MultiPortSwitch  Inputs=4
  Out1 : Outport
  wires:
  Constant10/1 -> Add/1
  Add/1 -> Multiport Switch/1
  Constant1/1 -> Multiport Switch/2
  Constant11/1 -> Multiport Switch/3
  Constant12/1 -> Multiport Switch/4
  Constant13/1 -> Multiport Switch/5
  In1/1 -> Add/2
  Multiport Switch/1 -> Out1/1

== system AssembledTEST1/Subsystem/Lateral//Directional Aerodynamics/getYLN/Subsystem ==
  In1 : Inport
  Add : Sum
  Get_sigma : Lookup  InputValues=side_data(1,:)  Table=side_data(2,:)
  Ground : Ground
  If : If  IfExpression=u1 < 0
  If Action Subsystem : Subsystem  TreatAsAtomicUnit=on
  If Action Subsystem1 : Subsystem  TreatAsAtomicUnit=on
  get_cpf : Fcn  Expr=(0.060 * (1 -cos(u(1))) )+( 0.444 * sin(u(1)));
  Out1 : Outport
  wires:
  Get_sigma/1 -> If Action Subsystem/1(In1)
  If/2 -> If Action Subsystem/Action
  If/1 -> If Action Subsystem1/Action
  Ground/1 -> If Action Subsystem1/1(In1)
  get_cpf/1 -> If/1, Get_sigma/1
  If Action Subsystem1/1(Out1) -> Add/1
  If Action Subsystem/1(Out1) -> Add/2
  In1/1 -> get_cpf/1
  Add/1 -> Out1/1

== system AssembledTEST1/Subsystem/Lateral//Directional Aerodynamics/getYLN/get_l_xi ==
  In3 : Inport
  In2 : Inport  Port=2
  In1 : Inport  Port=3
  Add1 : Sum  Inputs=+-
  Get_l_xi : Lookup  InputValues=ld_data(:,1)  Table=ld_data(:,12)
  Product1 : Product  RndMeth=Zero
  Out1 : Outport
  wires:
  Get_l_xi/1 -> Product1/1
  Add1/1 -> Product1/2
  In1/1 -> Get_l_xi/1
  Product1/1 -> Out1/1
  In2/1 -> Add1/1
  In3/1 -> Add1/2

== system AssembledTEST1/Subsystem/Lateral//Directional Aerodynamics/getYLN/get_n_xi ==
  In1 : Inport
  In2 : Inport  Port=2
  In3 : Inport  Port=3
  In4 : Inport  Port=4
  In5 : Inport  Port=5
  Add1 : Sum  Inputs=-+
  Add2 : Sum  Inputs=+-
  Add3 : Sum
  Embedded MATLAB Function : MATLAB Function  TreatAsAtomicUnit=on
  Gain : Gain  Gain=-1
  Get_Gi : Lookup  InputValues=ld_data(:,1)  Table=ld_data(:,13)
  Get_Go : Lookup  InputValues=ld_data(:,1)  Table=ld_data(:,14)
  Get_L_xi : Lookup  InputValues=ld_data(:,1)  Table=ld_data(:,12)
  Mux{,1..3} (4 alike) : Mux  Inputs=2
  Product : Product  RndMeth=Zero
  Product1 : Product  RndMeth=Zero
  Product2 : Product  Inputs=3  RndMeth=Zero
  average : Fcn  Expr=0.5*(u(1)+u(2))
  get_F_part : Fcn  Expr=(0.498 * u(1)) + 2.8 + (18 * u(2))
  get_Fi : Fcn  Expr=0.00770*u(2)-u(1)
  get_Fo : Fcn  Expr=0.00715*u(1)-u(2)
  r2d : Fcn  Expr=u(1)*180/pi
  Out1 : Outport
  wires:
  In3/1 -> Get_Go/1, Get_Gi/1, Get_L_xi/1
  Gain/1 -> [xi_s]
  [xi_s] -> Embedded MATLAB Function/1(xi_s)
  [xi_p] -> Embedded MATLAB Function/2(xi_p)
  [xi_s] -> Mux/1
  [xi_p] -> Mux/2
  [xi_s] -> Add1/1
  [xi_p] -> Add1/2
  Mux/1 -> average/1
  Add1/1 -> r2d/1
  r2d/1 -> Mux1/1
  Mux1/1 -> get_F_part/1
  Get_Gi/1 -> Product/1
  In4/1 -> Product1/1, Product/2
  Get_Go/1 -> Product1/2
  Mux2/1 -> get_Fi/1
  Product/1 -> Mux2/1
  get_F_part/1 -> Mux2/2, Mux3/1
  Mux3/1 -> get_Fo/1
  Product1/1 -> Mux3/2
  get_Fi/1 -> Add2/1
  get_Fo/1 -> Add2/2
  Get_L_xi/1 -> Product2/1
  Add2/1 -> Product2/2
  average/1 -> Product2/3
  Embedded MATLAB Function/1(C_np) -> Add3/1
  Product2/1 -> Add3/2
  In1/1 -> Gain/1
  Add3/1 -> Out1/1
  In2/1 -> [xi_p]
  In5/1 -> Mux1/2

== system AssembledTEST1/Subsystem/Longitudinal Aerodynamics/Get Drag/get_CDvt ==
  CLt : Inport
  Mach : Inport  Port=2
  Add5 : Sum
  Constant2 : Constant  Value=piAt
  Divide : Product  Inputs=*/
  Fcn : Fcn  Expr=u(1)^2
  Product4 : Product  RndMeth=Zero
  Product5 : Product  RndMeth=Zero
  get_1+d : Lookup  InputValues=vortex_drag_factors(:,1)  Table=vortex_drag_factors(:,3)
  get_K1 : Lookup  InputValues=vortex_drag_factors(:,1)  Table=vortex_drag_factors(:,2)
  CDvt : Outport
  wires:
  get_K1/1 -> Product4/1
  Constant2/1 -> Product4/2, Divide/2
  Product4/1 -> Add5/1
  get_1+d/1 -> Add5/2
  Add5/1 -> Divide/1
  Fcn/1 -> Product5/1
  Divide/1 -> Product5/2
  Mach/1 -> get_K1/1, get_1+d/1
  CLt/1 -> Fcn/1
  Product5/1 -> CDvt/1

== system AssembledTEST1/Subsystem/Longitudinal Aerodynamics/Get Drag/get_CDvw ==
  aoa_w : Inport
  flap : Inport  Port=2
  CLw : Inport  Port=3
  Mach : Inport  Port=4
  Add4 : Sum  Inputs=+++
  Constant2 : Constant  Value=piAw
  Divide : Product  Inputs=*/
  Fcn1 : Fcn  Expr=u(1)^2
  Fcn2 : Fcn  Expr=u(1)^2
  Product3 : Product  RndMeth=Zero
  Product4 : Product  RndMeth=Zero
  Product5 : Product  Inputs=3  RndMeth=Zero
  get_CL1 : Sum  Inputs=+-
  get_DelCL0tw : Subsystem
  get_k1 : Lookup2D  RowIndex=aw_ords  ColumnIndex=Mach_ords  Table=k_data
  get_k1f : Lookup  InputValues=k1f_data(:,1)  Table=k1f_data(:,2)
  get_kf : Subsystem
  r2d : Gain  Gain=180/pi
  CDvw : Outport
  wires:
  get_DelCL0tw/1(DelCL0tw) -> get_CL1/2, Fcn2/1, Product5/2
  get_CL1/1 -> Fcn1/1, Product5/3
  Fcn2/1 -> Product3/1
  get_kf/1(kf) -> Product3/2
  Fcn1/1 -> Product4/1
  get_k1/1 -> Product4/2
  get_k1f/1 -> Product5/1
  Product5/1 -> Add4/1
  Product4/1 -> Add4/2
  Product3/1 -> Add4/3
  Add4/1 -> Divide/1
  Constant2/1 -> Divide/2
  flap/1 -> get_DelCL0tw/1(flap), get_kf/1(flap)
  Mach/1 -> get_DelCL0tw/2(Mach), get_kf/2(Mach), get_k1/2
  aoa_w/1 -> get_k1f/1, r2d/1
  Divide/1 -> CDvw/1
  CLw/1 -> get_CL1/1
  r2d/1 -> get_k1/1

== system AssembledTEST1/Subsystem/Longitudinal Aerodynamics/Get Drag/get_D0//q_flap ==
  flap : Inport
  Constant1 : Constant  Value=0
  Constant2 : Constant  Value=D0q_10
  Constant3 : Constant  Value=D0q_20
  Constant4 : Constant  Value=D0q_35
  Multiport Switch : MultiPortSwitch  Inputs=4
  D0q_flap : Outport
  wires:
  Constant1/1 -> Multiport Switch/2
  Constant2/1 -> Multiport Switch/3
  Constant3/1 -> Multiport Switch/4
  Constant4/1 -> Multiport Switch/5
  flap/1 -> Multiport Switch/1
  Multiport Switch/1 -> D0q_flap/1

== system AssembledTEST1/Subsystem/Longitudinal Aerodynamics/Get Fin XZM/Get XZM ==
  L : Inport
  D : Inport  Port=2
  alpha : Inport  Port=3
  M0 : Inport  Port=4
  x : Inport  Port=5
  z : Inport  Port=6
  Add : Sum  Inputs=--
  Add1 : Sum  Inputs=+-
  Add2 : Sum  Inputs=-++
  Product{,1..5} (6 alike) : Product  RndMeth=Zero
  Trigonometric Function : Trigonometry
  Trigonometric Function1 : Trigonometry  Operator=cos
  X : Outport
  Z : Outport  Port=2
  M : Outport  Port=3
  wires:
  alpha/1 -> Trigonometric Function/1, Trigonometric Function1/1
  L/1 -> Product1/1, Product/1
  Trigonometric Function1/1 -> Product/2, Product2/1
  Trigonometric Function/1 -> Product1/2, Product3/1
  D/1 -> Product3/2, Product2/2
  Add/1 -> Product4/1, Z/1
  Product/1 -> Add/1
  Product3/1 -> Add/2
  Product1/1 -> Add1/1
  Product2/1 -> Add1/2
  Add1/1 -> Product5/1, X/1
  Product4/1 -> Add2/1
  Product5/1 -> Add2/2
  x/1 -> Product4/2
  Add2/1 -> M/1
  z/1 -> Product5/2
  M0/1 -> Add2/3

== system AssembledTEST1/Subsystem/Longitudinal Aerodynamics/Get Fuselage XZM/Subsystem ==
  In2 : Inport
  In1 : Inport  Port=2
  Add : Sum
  Constant : Constant
  Multiport Switch : MultiPortSwitch  Inputs=4
  get_fmf_10 : Lookup  InputValues=fmf_data(:,1)  Table=fmf_data(:,2)
  get_fmf_20 : Lookup  InputValues=fmf_data(:,1)  Table=fmf_data(:,3)
  get_fmf_35 : Lookup  InputValues=fmf_data(:,1)  Table=fmf_data(:,4)
  get_fmf_clean : Lookup  InputValues=fmc_data(:,1)  Table=fmc_data(:,2)
  Out1 : Outport
  wires:
  In1/1 -> get_fmf_clean/1, get_fmf_10/1, get_fmf_20/1, get_fmf_35/1
  In2/1 -> Add/1
  Constant/1 -> Add/2
  Add/1 -> Multiport Switch/1
  Multiport Switch/1 -> Out1/1
  get_fmf_clean/1 -> Multiport Switch/2
  get_fmf_10/1 -> Multiport Switch/3
  get_fmf_20/1 -> Multiport Switch/4
  get_fmf_35/1 -> Multiport Switch/5

== system AssembledTEST1/Subsystem/Longitudinal Aerodynamics/Get Nacelles XZM/Get XZM ==
  L : Inport
  D : Inport  Port=2
  alpha : Inport  Port=3
  M0 : Inport  Port=4
  x : Inport  Port=5
  z : Inport  Port=6
  Add : Sum  Inputs=--
  Add1 : Sum  Inputs=+-
  Add2 : Sum  Inputs=-++
  Product{,1..5} (6 alike) : Product  RndMeth=Zero
  Trigonometric Function : Trigonometry
  Trigonometric Function1 : Trigonometry  Operator=cos
  X : Outport
  Z : Outport  Port=2
  M : Outport  Port=3
  wires:
  alpha/1 -> Trigonometric Function/1, Trigonometric Function1/1
  L/1 -> Product1/1, Product/1
  Trigonometric Function1/1 -> Product/2, Product2/1
  Trigonometric Function/1 -> Product1/2, Product3/1
  D/1 -> Product3/2, Product2/2
  Add/1 -> Product4/1, Z/1
  Product/1 -> Add/1
  Product3/1 -> Add/2
  Product1/1 -> Add1/1
  Product2/1 -> Add1/2
  Add1/1 -> Product5/1, X/1
  Product4/1 -> Add2/1
  Product5/1 -> Add2/2
  x/1 -> Product4/2
  Add2/1 -> M/1
  z/1 -> Product5/2
  M0/1 -> Add2/3

== system AssembledTEST1/Subsystem/Longitudinal Aerodynamics/Get Nacelles XZM/Subsystem ==
  In2 : Inport
  In1 : Inport  Port=2
  Add : Sum
  Constant : Constant
  Gain : Gain  Gain=2
  Multiport Switch : MultiPortSwitch  Inputs=4
  get_fmn_10 : Lookup  InputValues=fmn_data(:,1)  Table=fmn_data(:,2)
  get_fmn_20 : Lookup  InputValues=fmn_data(:,1)  Table=fmn_data(:,3)
  get_fmn_35 : Lookup  InputValues=fmn_data(:,1)  Table=fmn_data(:,4)
  get_fmn_clean : Lookup  InputValues=fmc_data(:,1)  Table=fmc_data(:,3)
  Out1 : Outport
  wires:
  In1/1 -> get_fmn_10/1, get_fmn_clean/1, get_fmn_20/1, get_fmn_35/1
  In2/1 -> Add/1
  Constant/1 -> Add/2
  Add/1 -> Multiport Switch/1
  get_fmn_clean/1 -> Multiport Switch/2
  get_fmn_10/1 -> Multiport Switch/3
  get_fmn_20/1 -> Multiport Switch/4
  get_fmn_35/1 -> Multiport Switch/5
  Multiport Switch/1 -> Gain/1
  Gain/1 -> Out1/1

== system AssembledTEST1/Subsystem/Longitudinal Aerodynamics/Get Tail XZM/Get XZM ==
  L : Inport
  D : Inport  Port=2
  alpha : Inport  Port=3
  M0 : Inport  Port=4
  x : Inport  Port=5
  z : Inport  Port=6
  Add : Sum  Inputs=--
  Add1 : Sum  Inputs=+-
  Add2 : Sum  Inputs=-++
  Product{,1..5} (6 alike) : Product  RndMeth=Zero
  Trigonometric Function : Trigonometry
  Trigonometric Function1 : Trigonometry  Operator=cos
  X : Outport
  Z : Outport  Port=2
  M : Outport  Port=3
  wires:
  alpha/1 -> Trigonometric Function/1, Trigonometric Function1/1
  L/1 -> Product1/1, Product/1
  Trigonometric Function1/1 -> Product/2, Product2/1
  Trigonometric Function/1 -> Product1/2, Product3/1
  D/1 -> Product3/2, Product2/2
  Add/1 -> Product4/1, Z/1
  Product/1 -> Add/1
  Product3/1 -> Add/2
  Product1/1 -> Add1/1
  Product2/1 -> Add1/2
  Add1/1 -> Product5/1, X/1
  Product4/1 -> Add2/1
  Product5/1 -> Add2/2
  x/1 -> Product4/2
  Add2/1 -> M/1
  z/1 -> Product5/2
  M0/1 -> Add2/3
